simulink model "ADRC_Pure_Pursuit"  (R2023a)
settings: Solver=ode4  StartTime=0.0  StopTime=100  RelTol=1e-3
values from neighbouring files (symbols this model uses):
  Caf = 140000    [ADRC_PP.m]    (also in ADRC_Pure_Pursuit.m)
  Izz = 1000    [ADRC_PP.m]    (also in ADRC_Pure_Pursuit.m)
  K1 = 48    [ADRC_PP.m]    (also in ADRC_Pure_Pursuit.m = 24)
  K2 = 320    [ADRC_PP.m]    (also in ADRC_Pure_Pursuit.m = 80)
  la_ratio = 0.6    [ADRC_PP.m]    (also in ADRC_Pure_Pursuit.m)
  lf = 1.63886    [ADRC_PP.m]    (also in ADRC_Pure_Pursuit.m)
  lr = 1.248156    [ADRC_PP.m]    (also in ADRC_Pure_Pursuit.m)
  observer_discrete = c2d(observer, T)    [ADRC_PP.m]    (also in ADRC_Pure_Pursuit.m)
  X_path = linspace(start_point, end_point, 1000)    [ADRC_PP.m]    (also in ADRC_Pure_Pursuit.m)
  Y_path = polyval(poly_path, X_path)    [ADRC_PP.m]    (also in ADRC_Pure_Pursuit.m)
libraries: simulink x1, autolibshared x1
settings Model: Creator=adlink  LastModifiedBy=adlink

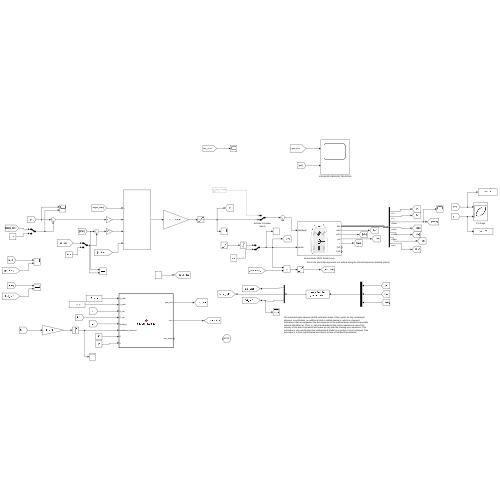
[thumbnail: Simulink's stored preview of the top-level diagram]
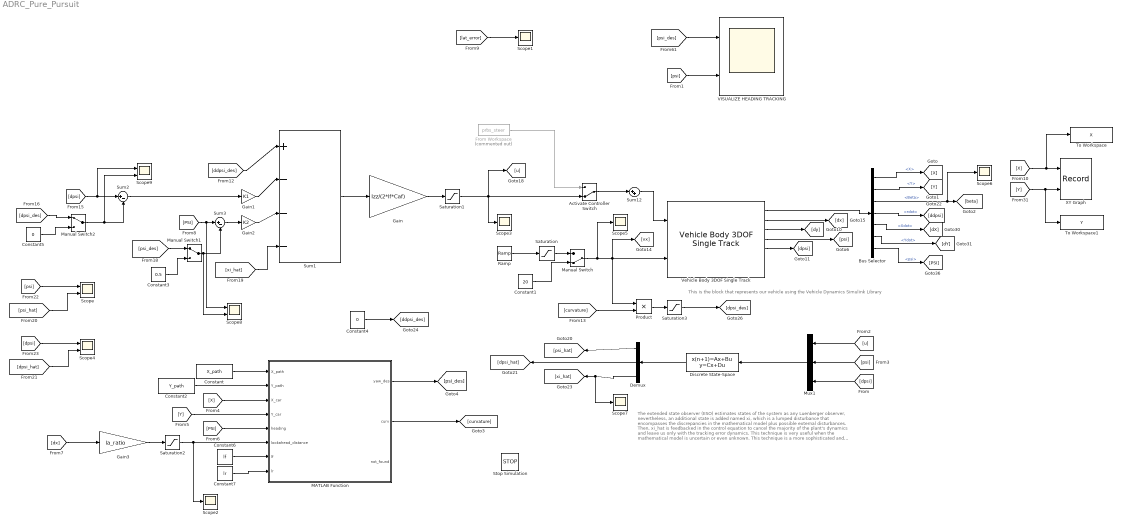
== system ADRC_Pure_Pursuit ==
  note: The extended state observer (ESO) estimates states of the system as any Luenberger observer, nevertheless, an additional state is added named xi, which is a lumped disturbance that encompasses the discrepancies in the mathematical model plus possible external disturbances. Then, xi_hat is feedbacked in the control equation to cancel the majority of the plant's dynamics and leave us only with the tracking error dynamics. This technique is very useful when the mathematical model is uncertain or even unknown. This technique is a more sophisticated and robust version of feedback linearization.
  note: This is the block that represents our vehicle using the Vehicle Dynamics Simulink Library
  Activate Controller Switch : ManualSwitch  CurrentSetting=0
  Bus Selector : BusSelector  OutputSignals=InertFrm.Cg.Disp.X,InertFrm.Cg.Disp.Y,BdyFrm.Cg.Ang.Beta,BdyFrm.Cg.AngAcc.rdot,InertFrm.Cg.Vel.Xdot,InertFrm.Cg.Vel.Ydot,InertFrm.Cg.Ang.psi
  Constant : Constant  Value=X_path
  Constant1 : Constant  Value=20
  Constant2 : Constant  Value=Y_path
  Constant3 : Constant  Value=0.5
  Constant4 : Constant  Value=0
  Constant5 : Constant  Value=0
  Constant6 : Constant  Value=lf
  Constant7 : Constant  Value=lr
  Demux : Demux  Outputs=3
  Discrete State-Space : DiscreteStateSpace  A=observer_discrete.A  B=observer_discrete.B  C=observer_discrete.C  D=observer_discrete.D  SampleTime=0.01
  From Workspace : FromWorkspace  Commented=on  VariableName=prbs_steer
  Gain : Gain  Gain=Izz/(2*lf*Caf)
  Gain1 : Gain  Gain=K1
  Gain2 : Gain  Gain=K2
  Gain3 : Gain  Gain=la_ratio
  MATLAB Function : MATLAB Function  TreatAsAtomicUnit=on
  Manual Switch : ManualSwitch  CurrentSetting=0
  Manual Switch1 : ManualSwitch
  Manual Switch2 : ManualSwitch
  Mux1 : Mux  Inputs=3
  Product : Product
  Ramp : simulink/Sources/Ramp  slope=1.2  start=1  InitialOutput=5
  Saturation : Saturate  UpperLimit=10  LowerLimit=-20
  Saturation1 : Saturate
  Saturation2 : Saturate  UpperLimit=50  LowerLimit=10
  Saturation3 : Saturate
  Scope{,4,8..9} (4 alike) : Scope  NumInputPorts=2
  Scope{1..3,5..7} (6 alike) : Scope
  Stop Simulation : Stop
  Sum1 : Sum  Inputs=|+---
  Sum12 : Sum  Inputs=|++
  Sum2 : Sum  Inputs=|+-
  Sum3 : Sum  Inputs=|+-
  To Workspace : ToWorkspace  VariableName=X  SaveFormat=Timeseries  SampleTime=0.01
  To Workspace1 : ToWorkspace  VariableName=Y  SaveFormat=Timeseries  SampleTime=0.01
  VISUALIZE HEADING TRACKING : Scope  NumInputPorts=2
  Vehicle Body 3DOF Single Track : autolibshared/Vehicle Body 3DOF Single Track  trackMode=Single (bicycle)  inputMode=External longitudinal velocity  frontSteerMode=on  rearSteerMode=off  windMode=off  muMode=off  extFMode=off  extMMode=off  htchFMode=off  htchMMode=off  extXo=off  extpsio=off  extxdoto=off  extro=off  extYo=off  extTamb=off  extydoto=off  aMode=2  NF=2  NR=2  m=630  a=1.723644  b=1.248156  h=0.35  dh=1  hh=0.2  X_o=0  xdot_o=0  CalphaMode=off  sigmaMode=on  d=0  hl=0  w=[1.4,1.4]  Cy_f=140000  Cy_r=140000  sigma_f=.1  sigma_r=.1  alpha_f_brk=[-.1 .1]  Cy_f_data=[-9e3 9e3]  alpha_r_brk=[-.1 .1]  Cy_r_data=[-9e3 9e3]  Y_o=0  ydot_o=0  Izz=1000  psi_o=0  r_o=0  Af=0.5  Cd=.3  Cl=.1  Cpm=.1  beta_w=[0 0.01:0.01:0.3]  Cs=[0 0.01:0.01:0.3]  Cym=[0 1e-6:0.01:0.3]  Pabs=101325  Tair=273  g=9.81  mu=1  xdot_tol=.01  Fznom=6200  Fxtire_sat=7e4  Fytire_sat=7e4  longOff=0  latOff=0  vertOff=0  wrapAng=off
  XY Graph : Record  FileSettingsInternal="{\"entries\":[{\"content\":{\"excelSettings\":{\"content\":{},\"type\":\"Streamout.ExcelSettings\"}},\"type\":\"Streamout.FileSettingStorage\",\"uuid\":\"\"}],\"packageUris\":[\"http:\\/\\/schema.mathworks.com\\/mf0\\/streamout_blocks\\/R2020a\"],\"version\":\"1.0\"}"  Layout=[1 1]  SignalsInternal="{\"entries\":[{\"content\":{\"signals\":[{\"content\":{\"blockPath\":[],\"dimensions\":[1],\"domain\":\"\",\"lineColor\":\"#a2142f\",\"port\":1,\"sid\":[\"\"],\"signalID\":2481,\"signalName\":\"From10\"},\"type\":\"RecordBlkView.Signal\",\"uuid\":\"\"},{\"content\":{\"blockPath\":[],\"dimensions\":[1],\"domain\":\"\",\"lineColor\":\"#139fff\",\"plots\":[1],\"port\":2,\"sid\":[\"\"],\"signalID\":2485,\"signalName\":\"From31\"},\"type\":\"RecordBlkView.Signal\",\"uuid\":\"\"}]},\"type\":\"RecordBlkView.InputSignals\",\"uuid\":\"\"}],\"packageUris\":[\"http:\\/\\/schema.mathworks.com\\/mf0\\/streamout_blocks\\/R2020a\"],\"version\":\"1.0\"}"  VisualizationBindings="{\"xyplotplugin\":{\"info\":[{\"series\":[{\"bindingParametersList\":[{\"parameter\":\"Y-Axis\",\"signalID\":2485,\"signalName\":\"From31\"}],\"seriesID\":44628}],\"subplotID\":1}]}}"  CompatibilityTag=XY
  wires:
  [psi_hat] -> Scope/2
  Bus Selector/2 -> [Y]  "<Y>"
  [psi] -> Scope/1
  [psi_des] -> Manual Switch1/1
  Vehicle Body 3DOF Single Track/5 -> [dpsi]
  Vehicle Body 3DOF Single Track/2 -> [dx]
  Bus Selector/1 -> [X]  "<X>"
  [lat_error] -> Scope1/1
  [psi] -> Mux1/2
  [xi_hat] -> Sum1/4
  Sum12/1 -> Vehicle Body 3DOF Single Track/1
  Saturation1/1 -> Activate Controller Switch/2, Scope3/1, [u]
  Bus Selector/6 -> [dY]  "<Ydot>"
  Vehicle Body 3DOF Single Track/4 -> [psi]
  [X] -> To Workspace/1, XY Graph/1
  Gain/1 -> Saturation1/1
  Vehicle Body 3DOF Single Track/3 -> [dy]
  Bus Selector/5 -> [dX]  "<Xdot>"
  [dpsi_des] -> Manual Switch2/1
  Constant3/1 -> Manual Switch1/2
  Manual Switch/1 -> Scope5/1, Product/1, Vehicle Body 3DOF Single Track/2, [vx]
  Demux/1 -> [psi_hat]
  Saturation/1 -> Manual Switch/1
  Bus Selector/4 -> [ddpsi]  "<rdot>"
  From Workspace/1 -> Activate Controller Switch/1
  Constant4/1 -> [ddpsi_des]
  [dpsi] -> Mux1/3
  [psi] -> VISUALIZE HEADING TRACKING/2
  Sum2/1 -> Gain1/1
  [dpsi] -> Scope4/1
  Gain1/1 -> Sum1/2
  Ramp/1 -> Saturation/1
  Bus Selector/7 -> [PSI]  "<psi>"
  [Y] -> To Workspace1/1, XY Graph/2
  Constant1/1 -> Manual Switch/2
  [curvature] -> Product/2
  Manual Switch1/1 -> Scope8/2, Sum3/2
  Bus Selector/3 -> Scope6/1, [beta]  "<Beta>"
  Vehicle Body 3DOF Single Track/1 -> Bus Selector/1
  Constant5/1 -> Manual Switch2/2
  Sum1/1 -> Gain/1
  Gain2/1 -> Sum1/3
  [PSI] -> Scope8/1, Sum3/1
  Demux/2 -> [dpsi_hat]
  Manual Switch2/1 -> Scope9/2, Sum2/2
  Activate Controller Switch/1 -> Sum12/1
  Demux/3 -> Scope7/1, [xi_hat]
  [u] -> Mux1/1
  [dpsi_hat] -> Scope4/2
  [psi_des] -> VISUALIZE HEADING TRACKING/1
  [ddpsi_des] -> Sum1/1
  [dpsi] -> Scope9/1, Sum2/1
  Sum3/1 -> Gain2/1
  Constant/1 -> MATLAB Function/1(X_path)
  Constant2/1 -> MATLAB Function/2(Y_path)
  [X] -> MATLAB Function/3(X_car)
  [Y] -> MATLAB Function/4(Y_car)
  [PSI] -> MATLAB Function/5(heading)
  Gain3/1 -> Saturation2/1
  [dx] -> Gain3/1
  MATLAB Function/1(yaw_des) -> [psi_des]
  Discrete State-Space/1 -> Demux/1
  Mux1/1 -> Discrete State-Space/1
  Saturation2/1 -> Scope2/1, MATLAB Function/6(lookahead_distance)
  Constant6/1 -> MATLAB Function/7(lf)
  Constant7/1 -> MATLAB Function/8(lr)
  MATLAB Function/2(curv) -> [curvature]
  Product/1 -> Saturation3/1
  Saturation3/1 -> [dpsi_des]

== matlab function ADRC_Pure_Pursuit/MATLAB Function ==
  data: yaw_des output; X_path input; Y_path input; X_car input; Y_car input; heading input; lookahead_distance input; lf input; lr input; curv output; not_found output
function [yaw_des, curv, not_found]  = get_des_heading(X_path, Y_path, X_car, Y_car, heading, lookahead_distance, lf, lr)

    la = lookahead_distance;
    
    % 1. Get global -> cog transform:
    
    Toc = [cos(heading), -sin(heading), 0, X_car; 
        sin(heading), cos(heading), 0, Y_car; 
        0, 0, 1, 0;
        0, 0, 0, 1];
    
    % P_tar_o = [X_path, Y_path, 0, 1]';
    % desired_path_point = inv(Toc)*P_tar_o;

    % 2. Iteratively find the lookahead distance point transforming global path
    % points to cog frame:
    best_match = 10000;
    best_match_point = [0, 0, 0, 1]';
    not_found = 1; 

    for i = 1:length(X_path)
        P_tar_o = [X_path(i), Y_path(i), 0, 1]'; % o subscript stands for global frame, c stands for car frame (cog)
        P_tar_c = inv(Toc)*P_tar_o; % Change for \ operator for faster inversion

        if (P_tar_c(1) > 0)
            euclidean_distance = sqrt(P_tar_c(1)^2 + P_tar_c(2)^2);
            if (abs(euclidean_distance - la) < abs(best_match - la))
                best_match = euclidean_distance;
                best_match_point = P_tar_c;
            end
            if (euclidean_distance > la-1 && euclidean_distance < la+1)
                not_found = 0;
                break;
            end
        else
            continue;
        end
    end

    if not_found == 1
        P_tar_c = best_match_point;
    else
        disp('FOUND')
    end
    
    % % Calculate heading angle to target waypoint:
    % yaw_targ = atan2(P_tar_c(2), P_tar_c(1)) + heading;
    % 
    % % Calculate lookahead curvature component for des_yaw:
    % yaw_adj = atan(la*curv);
    % disp(curv)

    alpha = atan2(P_tar_c(2), P_tar_c(1));
    curv = 2*sin(alpha) / la;

    % Finally, calculate the desired heading:
    yaw_des = atan(2*(lf+lr)*sin(alpha) / la) + heading;

    formatSpec = 'Y_tar, Yaw_adj %0.5f,%0.5f';
    %sprintf(formatSpec, yaw_targ, yaw_adj)
    % fprintf(['Yt: ' num2str(yaw_targ) 'Yadj: ' num2str(yaw_adj)]);
